simulink model "AM_detector_w_PLL_2020"  (R2023b)
settings: Solver=ode45  StartTime=0.0  StopTime=0.699999  RelTol=1e-3  EnableMultiTasking=on
PreLoadFcn:
  | Df=1;
  | W=900;
  | G=100;
libraries: dspfdesign x6, commsynccomp2 x1
settings Model: Creator=morelos_zaragoza  LastModifiedBy=14083
settings SolverCC: AlgebraicLoopSolver=TrustRegion
settings DataIOCC: LimitDataPoints=on  SaveFormat=Array  SignalLoggingSaveFormat=ModelDataLogs  ReturnWorkspaceOutputs=off
settings OptimizationCC: ExpressionDepthLimit=2147483647  InitFltsAndDblsToZero=on  LifeSpan=inf
settings DebuggingCC: SaveWithParameterizedLinksMsg=none  UnderspecifiedInitializationDetection=Classic  MergeDetectMultiDrivingBlocksExec=none  SignalResolutionControl=TryResolveAllWithWarning  SolverPrmCheckMsg=warning  MultiTaskDSMMsg=warning  MultiTaskCondExecSysMsg=none  FcnCallInpInsideContextMsg=warning  UnconnectedInputMsg=warning  UnconnectedOutputMsg=warning  UnconnectedLineMsg=warning  StateNameClashWarn=warning  SFUnexpectedBacktrackingDiag=warning  SFNoUnconditionalDefaultTransitionDiag=warning  SFExecutionAtInitializationDiag=none  ArithmeticOperatorsInVariantConditions=warning
settings HardwareCC: ProdBitPerPointer=32  ProdBitPerSizeT=32  ProdBitPerPtrDiffT=32  ProdLargestAtomicFloat=None  ProdIntDivRoundTo=Undefined  ProdEndianess=Unspecified  ProdWordSize=32  ProdHWDeviceType=32-bit Generic
settings ModelReferenceCC: EnableRefExpFcnMdlSchedulingChecks=on  PropagateSignalLabelsOutOfModel=off
settings SFSimCC: SimUseLocalCustomCode=off  CustomCodeUndefinedFunction=UseInterfaceOnly
settings RTWCC: RTWUseLocalCustomCode=off
settings CodeAppCC: StateflowObjectComments=on
settings GRTTargetCC: TargetFcnLib=ansi_tfl_tmw.mat  TargetLangStandard=C89/C90 (ANSI)  CombineOutputUpdateFcns=off  GRTInterface=on
settings ConfigComp: CovMetricSettings=dw  CovSaveCumulativeToWorkspaceVar=on  CovSaveSingleToWorkspaceVar=on  CovExternalEMLEnable=off

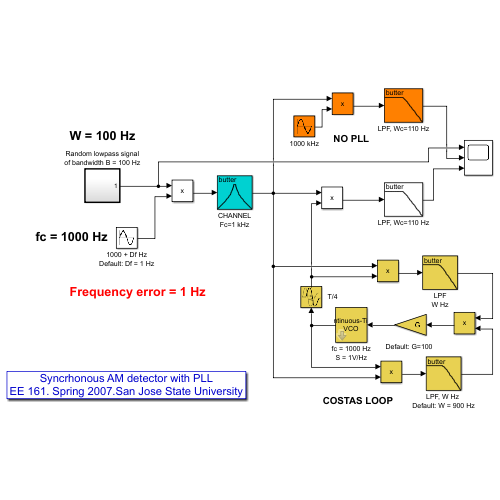
[thumbnail: Simulink's stored preview of the top-level diagram]
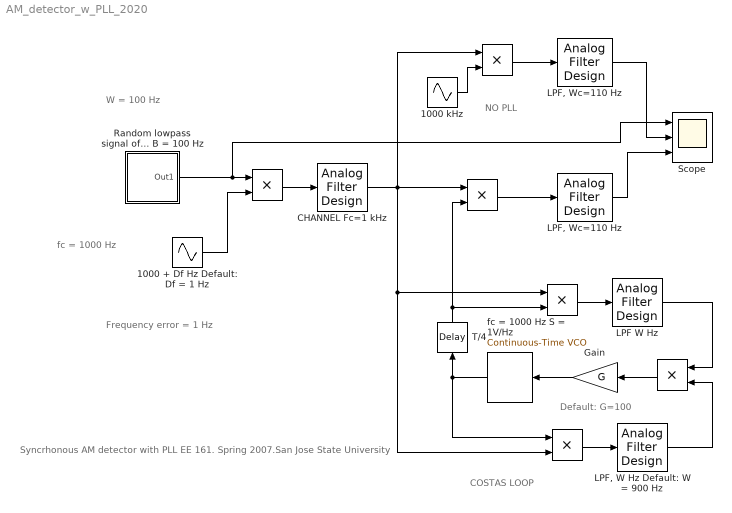
== system AM_detector_w_PLL_2020 ==
  note: W = 100 Hz
  note: Frequency error = 1 Hz
  note: Syncrhonous AM detector with PLL
      | EE 161. Spring 2007.San Jose State University
  note: COSTAS LOOP
  note: NO PLL
  note: Default: G=100
  note: fc = 1000 Hz
  " " : Product  RndMeth=Zero  SampleTime=1/100000
  "  " : Product  RndMeth=Zero  SampleTime=1/100000
  "   " : Product  RndMeth=Zero  SampleTime=1/100000
  "       " : Product  RndMeth=Zero
  "              " : Product  RndMeth=Zero
  "               " : Product  RndMeth=Zero  SampleTime=1/100000
  " LPF, Wc=110 Hz " : dspfdesign/Analog Filter Design  method=Butterworth  filttype=Lowpass  N=4  Wlo=2*pi*110  Whi=2*pi*110  Rp=2  Rs=60
  " T/4" : TransportDelay  DelayTime=(1/1000)*(1/4)  InitialOutput=1  BufferSize=1030  PadeOrder=1
  1000 + Df Hz Default: Df = 1 Hz : Sin  Frequency=2*pi*(1000+Df)  SampleTime=0
  1000 kHz : Sin  Frequency=2*pi*1000  SampleTime=0
  CHANNEL Fc=1 kHz : dspfdesign/Analog Filter Design  method=Butterworth  filttype=Bandpass  N=12  Wlo=2*pi*850  Whi=2*pi*1150  Rp=2  Rs=40
  Gain : Gain  Gain=G
  LPF W Hz : dspfdesign/Analog Filter Design  method=Butterworth  filttype=Lowpass  N=3  Wlo=2*pi*W  Whi=80  Rp=2  Rs=40
  "LPF, W Hz Default: W = 900 Hz" : dspfdesign/Analog Filter Design  method=Butterworth  filttype=Lowpass  N=3  Wlo=2*pi*W  Whi=80  Rp=2  Rs=40
  "LPF, Wc=110 Hz" : dspfdesign/Analog Filter Design  method=Butterworth  filttype=Lowpass  N=4  Wlo=2*pi*110  Whi=2*pi*110  Rp=2  Rs=60
  Random lowpass signal of bandwidth B = 100 Hz : Subsystem  TreatAsAtomicUnit=on
  Scope : Scope  NumInputPorts=3
  fc = 1000 Hz S = 1V/Hz : commsynccomp2/Continuous-Time VCO  Ac=1  Fc=1000  Kc=1  Ph=0
  wires:
  " "/1 -> LPF W Hz/1
  LPF W Hz/1 -> "               "/1
  Gain/1 -> fc = 1000 Hz S = 1V/Hz/1
  1000 + Df Hz Default: Df = 1 Hz/1 -> "  "/2
  Random lowpass signal of bandwidth B = 100 Hz/1(Out1) -> "  "/1, Scope/1
  "       "/1 -> "LPF, Wc=110 Hz"/1
  "  "/1 -> CHANNEL Fc=1 kHz/1
  CHANNEL Fc=1 kHz/1 -> "       "/1, "              "/1, " "/1, "   "/2
  "              "/1 -> " LPF, Wc=110 Hz "/1
  1000 kHz/1 -> "              "/2
  " LPF, Wc=110 Hz "/1 -> Scope/2
  "               "/1 -> Gain/1
  "LPF, W Hz Default: W = 900 Hz"/1 -> "               "/2
  "   "/1 -> "LPF, W Hz Default: W = 900 Hz"/1
  " T/4"/1 -> " "/2, "       "/2
  "LPF, Wc=110 Hz"/1 -> Scope/3
  fc = 1000 Hz S = 1V/Hz/1 -> " T/4"/1, "   "/1

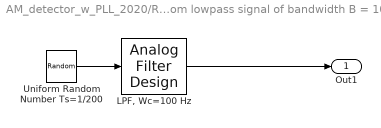
== system AM_detector_w_PLL_2020/Random lowpass signal of bandwidth B = 100 Hz ==
  "LPF, Wc=100 Hz" : dspfdesign/Analog Filter Design  method=Chebyshev II  filttype=Lowpass  N=22  Wlo=2*pi*100  Whi=2*pi*110  Rp=2  Rs=80
  Uniform Random Number Ts=1/200 : UniformRandomNumber  Seed=23453  SampleTime=1/200
  Out1 : Outport
  wires:
  Uniform Random Number Ts=1/200/1 -> "LPF, Wc=100 Hz"/1
  "LPF, Wc=100 Hz"/1 -> Out1/1
